simulink model "RCL_netzwerk_als_block"  (Simulink 7.7)
settings: Solver=ode45  StartTime=0.0  StopTime=15  RelTol=1e-3
values from neighbouring files (symbols this model uses):
  C = C(1:min(length(R),length(C)))    [InputMatFramer.m]    (also in OUT_OF_MEMORY.m; TIPS_TRICKS.m = strfind(C{1}, 'OptimetricsResult'))
undefined symbols (not defined in the file or in its folder): L, R1, R2
settings Model: Creator=mainster  LastModifiedBy=mainster
settings DebuggingCC: SolverPrmCheckMsg=none

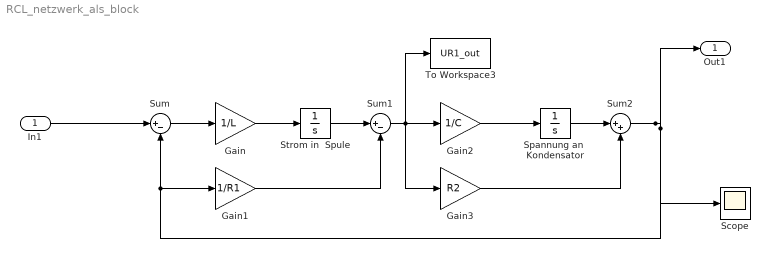
== system RCL_netzwerk_als_block ==
  In1 : Inport
  Gain : Gain  Gain=1/L
  Gain1 : Gain  Gain=1/R1
  Gain2 : Gain  Gain=1/C
  Gain3 : Gain  Gain=R2
  Scope : Scope
  Spannung an  Kondensator : Integrator
  Strom in  Spule : Integrator
  Sum : Sum  Inputs=|+-
  Sum1 : Sum  Inputs=|+-
  Sum2 : Sum  Inputs=|++
  To Workspace3 : ToWorkspace  VariableName=UR1_out  SampleTime=-1  SaveFormat=Structure
  Out1 : Outport
  wires:
  In1/1 -> Sum/1
  Sum/1 -> Gain/1
  Gain/1 -> Strom in  Spule/1
  Strom in  Spule/1 -> Sum1/1
  Sum1/1 -> Gain2/1, Gain3/1, To Workspace3/1
  Gain2/1 -> Spannung an  Kondensator/1
  Spannung an  Kondensator/1 -> Sum2/1
  Sum2/1 -> Scope/1, Sum/2, Gain1/1, Out1/1
  Gain1/1 -> Sum1/2
  Gain3/1 -> Sum2/2
